simulink model "interfacetypes_0003_fail"  (R2023b)
settings: Solver=VariableStepAuto  StartTime=0.0  StopTime=10.0  RelTol=1e-3
PostLoadFcn:
  | load BusObjectWS_File_fail.mat
settings Model: DataDictionary=correct_types.sldd  Creator=raarenst  LastModifiedBy=raarenst

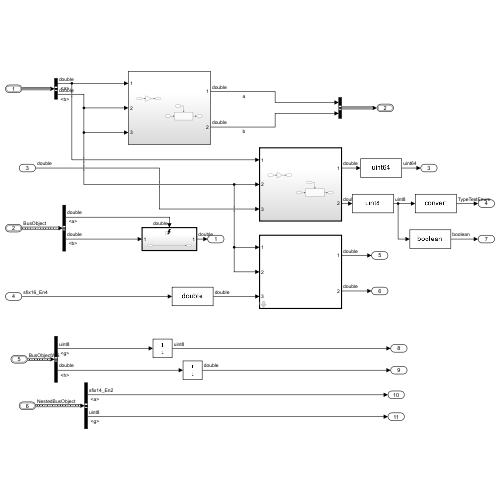
[thumbnail: Simulink's stored preview of the top-level diagram]
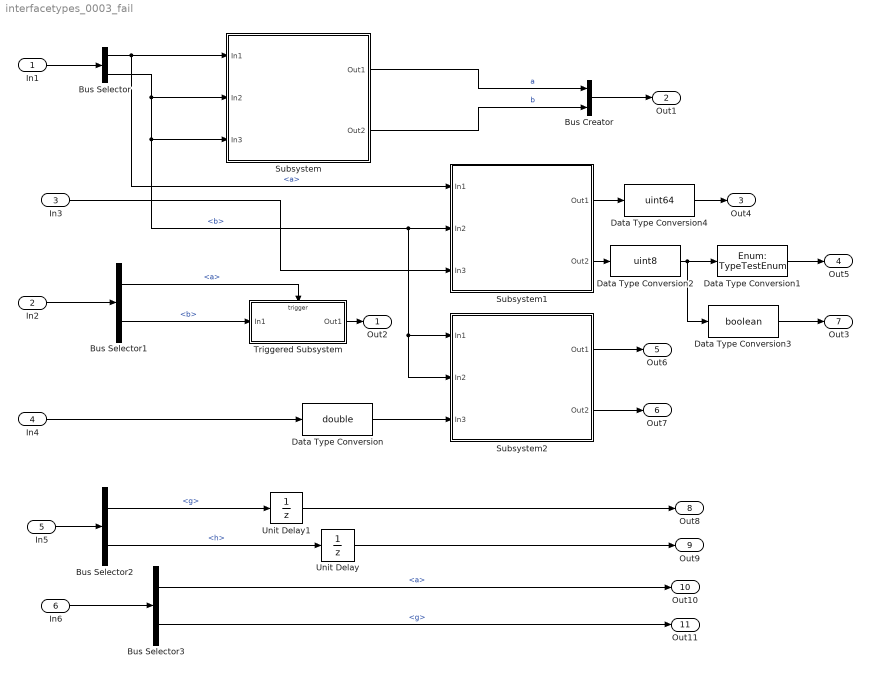
== system interfacetypes_0003_fail ==
  In1 : Inport  OutDataTypeStr=Bus: BusObject
  In2 : Inport  Port=2  OutDataTypeStr=Bus: BusObject  BusOutputAsStruct=on
  In3 : Inport  Port=3
  In4 : Inport  Port=4  OutDataTypeStr=fixdt(1,16,4)
  In5 : Inport  Port=5  OutDataTypeStr=Bus: BusObjectWS  BusOutputAsStruct=on
  In6 : Inport  Port=6  OutDataTypeStr=Bus: NestedBusObject  BusOutputAsStruct=on
  Bus Creator : BusCreator  Inputs=2
  Bus Selector : BusSelector  OutputSignals=a,b
  Bus Selector1 : BusSelector  OutputSignals=a,b
  Bus Selector2 : BusSelector  OutputSignals=g,h
  Bus Selector3 : BusSelector  OutputSignals=a1.a,a.g
  Data Type Conversion : DataTypeConversion  OutDataTypeStr=double  SaturateOnIntegerOverflow=off  RndMeth=Floor
  Data Type Conversion1 : DataTypeConversion  OutDataTypeStr=Enum: TypeTestEnum  SaturateOnIntegerOverflow=off  RndMeth=Floor
  Data Type Conversion2 : DataTypeConversion  OutDataTypeStr=uint8  SaturateOnIntegerOverflow=off  RndMeth=Floor
  Data Type Conversion3 : DataTypeConversion  OutDataTypeStr=boolean  SaturateOnIntegerOverflow=off  RndMeth=Floor
  Data Type Conversion4 : DataTypeConversion  OutDataTypeStr=uint64  SaturateOnIntegerOverflow=off  RndMeth=Floor
  Subsystem : Subsystem
  Subsystem1 : Subsystem  TreatAsAtomicUnit=on
  Subsystem2 : Subsystem  TreatAsAtomicUnit=on  mask{Parameter1=on}
  Triggered Subsystem : Subsystem  TreatAsAtomicUnit=on
  Unit Delay : UnitDelay  SampleTime=-1  HasFrameUpgradeWarning=on
  Unit Delay1 : UnitDelay  SampleTime=-1  HasFrameUpgradeWarning=on
  Out2 : Outport
  Out1 : Outport  Port=2  OutDataTypeStr=Bus: BusObject
  Out4 : Outport  Port=3
  Out5 : Outport  Port=4
  Out6 : Outport  Port=5
  Out7 : Outport  Port=6
  Out3 : Outport  Port=7
  Out8 : Outport  Port=8
  Out9 : Outport  Port=9
  Out10 : Outport  Port=10
  Out11 : Outport  Port=11
  wires:
  Bus Selector/1 -> Subsystem1/1(In1), Subsystem/1(In1)  "<a>"
  Triggered Subsystem/1(Out1) -> Out2/1
  Bus Selector1/2 -> Triggered Subsystem/1(In1)  "<b>"
  Bus Selector1/1 -> Triggered Subsystem/Trigger  "<a>"
  Bus Selector/2 -> Subsystem2/2(In2), Subsystem2/1(In1), Subsystem1/2(In2), Subsystem/3(In3), Subsystem/2(In2)  "<b>"
  Subsystem/1(Out1) -> Bus Creator/1  "a"
  Subsystem/2(Out2) -> Bus Creator/2  "b"
  Subsystem1/1(Out1) -> Data Type Conversion4/1
  Subsystem1/2(Out2) -> Data Type Conversion2/1
  Subsystem2/1(Out1) -> Out6/1
  Subsystem2/2(Out2) -> Out7/1
  In1/1 -> Bus Selector/1
  Bus Creator/1 -> Out1/1
  In2/1 -> Bus Selector1/1
  In3/1 -> Subsystem1/3(In3)
  In4/1 -> Data Type Conversion/1
  Data Type Conversion/1 -> Subsystem2/3(In3)
  Data Type Conversion1/1 -> Out5/1
  Data Type Conversion2/1 -> Data Type Conversion3/1, Data Type Conversion1/1
  Data Type Conversion3/1 -> Out3/1
  In5/1 -> Bus Selector2/1
  Bus Selector2/2 -> Unit Delay/1  "<h>"
  Unit Delay/1 -> Out9/1
  Bus Selector2/1 -> Unit Delay1/1  "<g>"
  Unit Delay1/1 -> Out8/1
  In6/1 -> Bus Selector3/1
  Bus Selector3/1 -> Out10/1  "<a>"
  Bus Selector3/2 -> Out11/1  "<g>"
  Data Type Conversion4/1 -> Out4/1

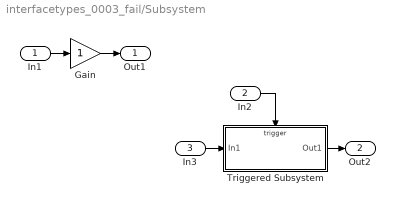
== system interfacetypes_0003_fail/Subsystem ==
  In1 : Inport
  In2 : Inport  Port=2
  In3 : Inport  Port=3
  Gain : Gain
  Triggered Subsystem : Subsystem  TreatAsAtomicUnit=on
  Out1 : Outport
  Out2 : Outport  Port=2
  wires:
  In3/1 -> Triggered Subsystem/1(In1)
  In1/1 -> Gain/1
  In2/1 -> Triggered Subsystem/Trigger
  Gain/1 -> Out1/1
  Triggered Subsystem/1(Out1) -> Out2/1

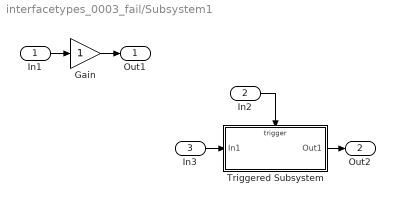
== system interfacetypes_0003_fail/Subsystem1 ==
  In1 : Inport
  In2 : Inport  Port=2
  In3 : Inport  Port=3
  Gain : Gain
  Triggered Subsystem : Subsystem  TreatAsAtomicUnit=on
  Out1 : Outport
  Out2 : Outport  Port=2
  wires:
  Triggered Subsystem/1(Out1) -> Out2/1
  Gain/1 -> Out1/1
  In2/1 -> Triggered Subsystem/Trigger
  In1/1 -> Gain/1
  In3/1 -> Triggered Subsystem/1(In1)

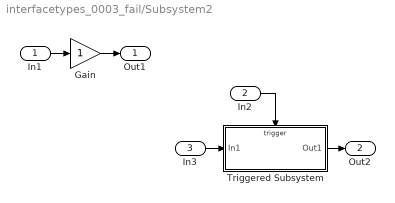
== system interfacetypes_0003_fail/Subsystem2 ==
  In1 : Inport
  In2 : Inport  Port=2
  In3 : Inport  Port=3
  Gain : Gain
  Triggered Subsystem : Subsystem  TreatAsAtomicUnit=on
  Out1 : Outport
  Out2 : Outport  Port=2
  wires:
  In3/1 -> Triggered Subsystem/1(In1)
  In1/1 -> Gain/1
  In2/1 -> Triggered Subsystem/Trigger
  Gain/1 -> Out1/1
  Triggered Subsystem/1(Out1) -> Out2/1

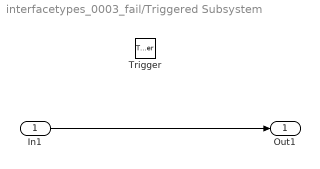
== system interfacetypes_0003_fail/Triggered Subsystem ==
  In1 : Inport
  Trigger : TriggerPort  VariantControl=(inherit)
  Out1 : Outport
  wires:
  In1/1 -> Out1/1

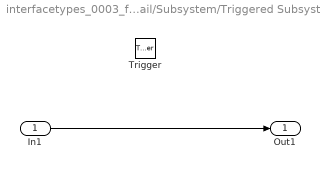
== system interfacetypes_0003_fail/Subsystem/Triggered Subsystem ==
  In1 : Inport
  Trigger : TriggerPort  VariantControl=(inherit)
  Out1 : Outport
  wires:
  In1/1 -> Out1/1

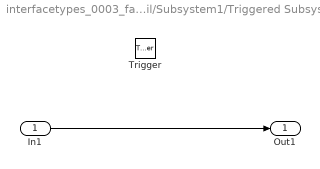
== system interfacetypes_0003_fail/Subsystem1/Triggered Subsystem ==
  In1 : Inport
  Trigger : TriggerPort  VariantControl=(inherit)
  Out1 : Outport
  wires:
  In1/1 -> Out1/1

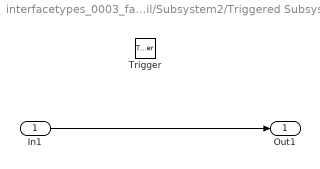
== system interfacetypes_0003_fail/Subsystem2/Triggered Subsystem ==
  In1 : Inport
  Trigger : TriggerPort  VariantControl=(inherit)
  Out1 : Outport
  wires:
  In1/1 -> Out1/1
